simulink library "truetime"  (Simulink 4.00)
undefined symbols (not defined in the file or in its folder): ttGetMsg2
settings Model: Creator=dan  LastModifiedBy=anton  ExtModeAutoUpdateStatusClock=off

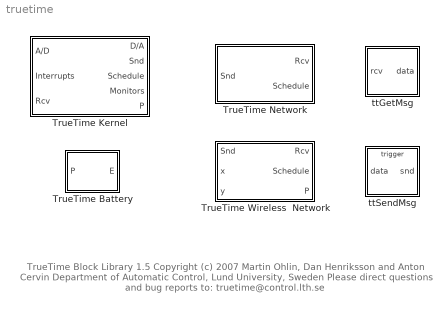
== system truetime ==
  note: TrueTime Block Library 1.5
      | Copyright (c) 2007
      | Martin Ohlin, Dan Henriksson and Anton Cervin
      | Department of Automatic Control, Lund University, Sweden
      | Please direct questions and bug reports to:  truetime@control.lth.se
  TrueTime Battery : Subsystem  mask{energy=1}
      mask prompts: energy "Watt seconds (Joule)"
      settings: RTWFcnNameOpts=Auto  RTWFileNameOpts=Auto
  TrueTime Kernel : Subsystem  mask{sfun=node_init, args=0, battery=off, clockdrift=0, clockoffset=0}
      mask prompts: sfun "Name of init function (MEX or MATLAB)"; args "Init function argument"; clockdrift "Clock drift"; clockoffset "Clock offset"
      settings: RTWFcnNameOpts=Auto  RTWFileNameOpts=Auto
      mask CallbackString: ||kernel_callback||
  TrueTime Network : Subsystem  mask(Real-Time Network){nwtype=CSMA/CD (Ethernet), nwnbr=1, nnodes=2, rate=10000000, minsize=512, lossprob=0, bandwidths=[0.5 0.5], slotsize=512, schedule=[1 1 2], memsize=80000, buftype=Common buffer, overflow=Retransmit}
      mask prompts: nwtype "Network type"; nwnbr "Network number"; nnodes "Number of nodes"; rate "Data rate (bits/s)"; minsize "Minimum frame size (bits)"; lossprob "Loss probability (0-1)"; bandwidths "Bandwidth allocations"; slotsize "Slotsize (bits)"; schedule "Cyclic schedule"; memsize "Total switch memory (bits)"; buftype "Switch buffer type"; overflow "Switch overflow behavior"
      settings: RTWFcnNameOpts=Auto  RTWFileNameOpts=Auto
      mask StyleString: popup(CSMA/CD (Ethernet)|CSMA/AMP (CAN)|Round Robin|FDMA|TDMA|Switched Ethernet),edit,edit,edit,edit,edit,edit,edit,edit,edit,popup(Common buffer|Symmetric output buffers),popup(Retransmit|Drop)
      mask CallbackString: network_callback||network_callback|network_callback|||network_callback|network_callback|network_callback|||
      mask Display: disp(nwnbr)
  TrueTime Wireless  Network : Subsystem  mask(Wireless Network){nwtype=802.11b (WLAN), nwnbr=1, nnodes=2, rate=800000, minsize=272, transpower=20, threshold=-48, pathloss=3.5, use_pathloss_function=off, pathloss_function=, acktimeout=0.00004, retrylimit=5, error_threshold=0.03}
      mask prompts: nwtype "Network type"; nwnbr "Network Number"; nnodes "Number of nodes"; rate "Data rate (bits/s)"; minsize "Minimum frame size (bits)"; transpower "Transmit power (dbm)"; threshold "Receiver signal threshold (dbm)"; pathloss "Pathloss exponent (1/distance^x)"; use_pathloss_function "Special pathloss function"; pathloss_function "Matlab pathloss function"; acktimeout "ACK timeout (s)"; retrylimit "Retry limit"; error_threshold "Error coding threshold"
      settings: RTWFcnNameOpts=Auto  RTWFileNameOpts=Auto
      mask StyleString: popup(802.11b (WLAN)|802.15.4 (ZigBee)),edit,edit,edit,edit,edit,edit,edit,checkbox,edit,edit,edit,edit
      mask CallbackString: wnetwork_callback||||||||pathloss_button||||
      mask Display: disp(nwnbr)
  ttGetMsg : Subsystem  TreatAsAtomicUnit=on  mask{network=1, receiver=1, trigger=off}
      mask prompts: network "network number"; receiver "receiver id"; trigger "trigger output"
      settings: RTWFcnNameOpts=Auto  RTWFileNameOpts=Auto
      mask CallbackString: ||getmsg_callback
  ttSendMsg : Subsystem  TreatAsAtomicUnit=on  mask{network=1, network_input=off, sender=1, sender_input=off, receiver=2, receiver_input=off, data=0, data_input=on, length=40, length_input=off, prio=1, priority_input=off, TriggerType=either}
      mask prompts: network "network number"; network_input "Add network number input port"; sender "sender id"; sender_input "Add sender id input port"; receiver "receiver id"; receiver_input "Add receiver id input port"; data_input "Add data input port"; length "data length (bits)"; length_input "Add length input port"; prio "priority (only used for prioritized networks)"; priority_input "Add priority input port"; TriggerType "Trigger type:"
      settings: RTWFcnNameOpts=Auto  RTWFileNameOpts=Auto
      mask StyleString: edit,checkbox,edit,checkbox,edit,checkbox,edit,checkbox,edit,checkbox,edit,checkbox,popup(rising|falling|either)
      mask CallbackString: |sendmsg_callback||sendmsg_callback||sendmsg_callback||sendmsg_callback||sendmsg_callback||sendmsg_callback|sendmsg_callback

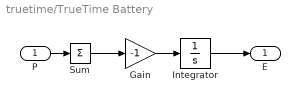
== system truetime/TrueTime Battery ==
  P : Inport  Port=1  LatchInput=off
  Gain : Gain  Gain=-1  Multiplication=Element-wise(K.*u)  SaturateOnIntegerOverflow=on
  Integrator : Integrator  ExternalReset=none  InitialConditionSource=internal  InitialCondition=energy  LimitOutput=on  UpperSaturationLimit=energy  LowerSaturationLimit=0  ShowSaturationPort=off  ShowStatePort=off  AbsoluteTolerance=auto
  Sum : Sum  Inputs=1  SaturateOnIntegerOverflow=on
  E : Outport  Port=1
  wires:
  Integrator/1 -> E/1
  Gain/1 -> Integrator/1
  P/1 -> Sum/1
  Sum/1 -> Gain/1

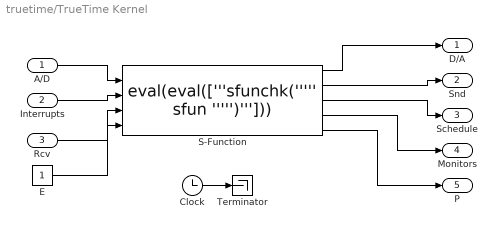
== system truetime/TrueTime Kernel ==
  A/D : Inport  Port=1  LatchInput=off
  Interrupts : Inport  Port=2  LatchInput=off
  Rcv : Inport  Port=3  LatchInput=off
  Clock : Clock
      settings: DisplayTime=off  Decimation=10
  E : Constant  Value=1
  S-Function : S-Function  FunctionName=eval(eval(['''sfunchk(''''' sfun ''''')''']))  Parameters=sfun, args, clockdrift, clockoffset  PortCounts=[]  SFunctionModules=''
  Terminator : Terminator
  D/A : Outport  Port=1
  Snd : Outport  Port=2
  Schedule : Outport  Port=3
  Monitors : Outport  Port=4
  P : Outport  Port=5
  wires:
  S-Function/5 -> P/1
  E/1 -> S-Function/4
  A/D/1 -> S-Function/1
  S-Function/2 -> Snd/1
  S-Function/1 -> D/A/1
  S-Function/3 -> Schedule/1
  S-Function/4 -> Monitors/1
  Interrupts/1 -> S-Function/2
  Rcv/1 -> S-Function/3
  Clock/1 -> Terminator/1

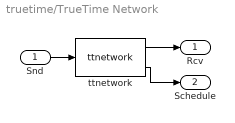
== system truetime/TrueTime Network ==
  Snd : Inport  Port=1  LatchInput=off
  ttnetwork : S-Function  FunctionName=ttnetwork  Parameters=nwtype,nwnbr,nnodes,rate,minsize,lossprob,bandwidths,slotsize,schedule,memsize,buftype,overflow  PortCounts=[]  SFunctionModules=''
  Rcv : Outport  Port=1
  Schedule : Outport  Port=2
  wires:
  ttnetwork/2 -> Schedule/1
  ttnetwork/1 -> Rcv/1
  Snd/1 -> ttnetwork/1

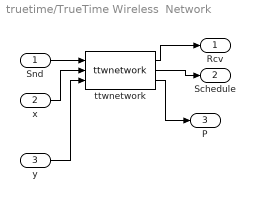
== system truetime/TrueTime Wireless  Network ==
  Snd : Inport  Port=1  LatchInput=off
  x : Inport  Port=2  LatchInput=off
  y : Inport  Port=3  LatchInput=off
  ttwnetwork : S-Function  FunctionName=ttwnetwork  Parameters=nwtype,nwnbr,nnodes,rate,minsize,transpower,threshold,pathloss,use_pathloss_function,pathloss_function,acktimeout,retrylimit,error_threshold  PortCounts=[]  SFunctionModules=''
  Rcv : Outport  Port=1
  Schedule : Outport  Port=2
  P : Outport  Port=3
  wires:
  ttwnetwork/3 -> P/1
  Snd/1 -> ttwnetwork/1
  ttwnetwork/1 -> Rcv/1
  ttwnetwork/2 -> Schedule/1
  x/1 -> ttwnetwork/2
  y/1 -> ttwnetwork/3

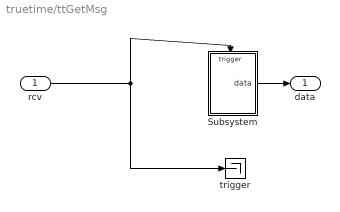
== system truetime/ttGetMsg ==
  rcv : Inport  Port=1  LatchInput=off
  Subsystem : Subsystem  TreatAsAtomicUnit=on
      settings: RTWFcnNameOpts=Auto  RTWFileNameOpts=Auto
  trigger : Terminator
  data : Outport  Port=1
  wires:
  Subsystem/1(data) -> data/1
  rcv/1 -> trigger/1, Subsystem/Trigger

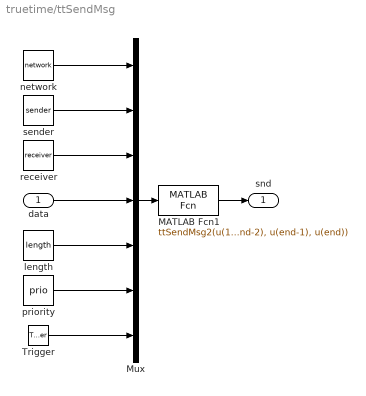
== system truetime/ttSendMsg ==
  data : Inport  Port=1  LatchInput=off
  Trigger : TriggerPort  TriggerType=either  ShowOutputPort=on  OutputDataType=auto
  MATLAB Fcn1 : MATLABFcn  MATLABFcn=ttSendMsg2(u(1), u(2), u(3), u(4:end-3), u(end-2), u(end-1), u(end))  OutputDimensions=-1  OutputSignalType=auto  Output1D=off
  Mux : Mux  Inputs=7
  length : Constant  Value=length
  network : Constant  Value=network
  priority : Constant  Value=prio
  receiver : Constant  Value=receiver
  sender : Constant  Value=sender
  snd : Outport  Port=1
  wires:
  MATLAB Fcn1/1 -> snd/1
  Mux/1 -> MATLAB Fcn1/1
  Trigger/1 -> Mux/7
  priority/1 -> Mux/6
  length/1 -> Mux/5
  data/1 -> Mux/4
  receiver/1 -> Mux/3
  sender/1 -> Mux/2
  network/1 -> Mux/1

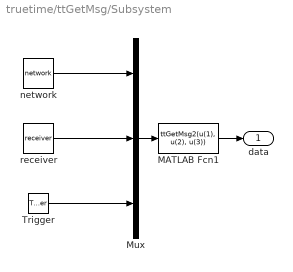
== system truetime/ttGetMsg/Subsystem ==
  Trigger : TriggerPort  TriggerType=either  ShowOutputPort=on  OutputDataType=auto
  MATLAB Fcn1 : MATLABFcn  MATLABFcn=ttGetMsg2(u(1), u(2), u(3))  OutputDimensions=-1  OutputSignalType=auto  Output1D=off
  Mux : Mux  Inputs=3
  network : Constant  Value=network
  receiver : Constant  Value=receiver
  data : Outport  Port=1
  wires:
  MATLAB Fcn1/1 -> data/1
  Mux/1 -> MATLAB Fcn1/1
  network/1 -> Mux/1
  receiver/1 -> Mux/2
  Trigger/1 -> Mux/3
